simulink model "Prueba_PID"  (R2023b)
settings: Solver=VariableStepAuto  StartTime=0.0  StopTime=10  RelTol=1e-3
values from neighbouring files (symbols this model uses):
  K1 = (2*Ts*Kp + Ki*Ts^2 + 2*Kd)/(2*Ts)    (= 55.639105)    [PID_SystemIdentification.m]
  K2 = (Ki*Ts^2 - 2*Ts*Kp - 4*Kd)/(2*Ts)    (= -94.547095)    [PID_SystemIdentification.m]
  K3 = (2*Kd)/(2*Ts)    (= 42.1)    [PID_SystemIdentification.m]
settings Model: Creator=PC  LastModifiedBy=Ruben

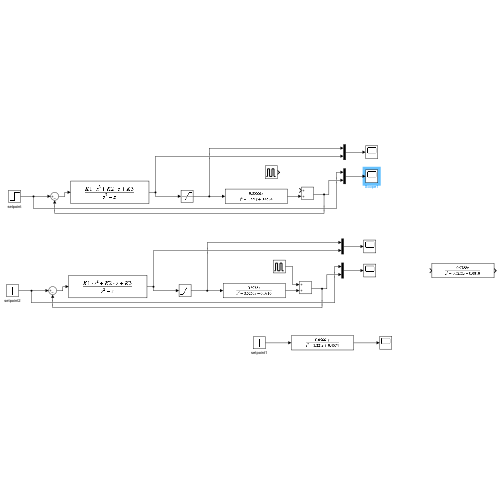
[thumbnail: Simulink's stored preview of the top-level diagram]
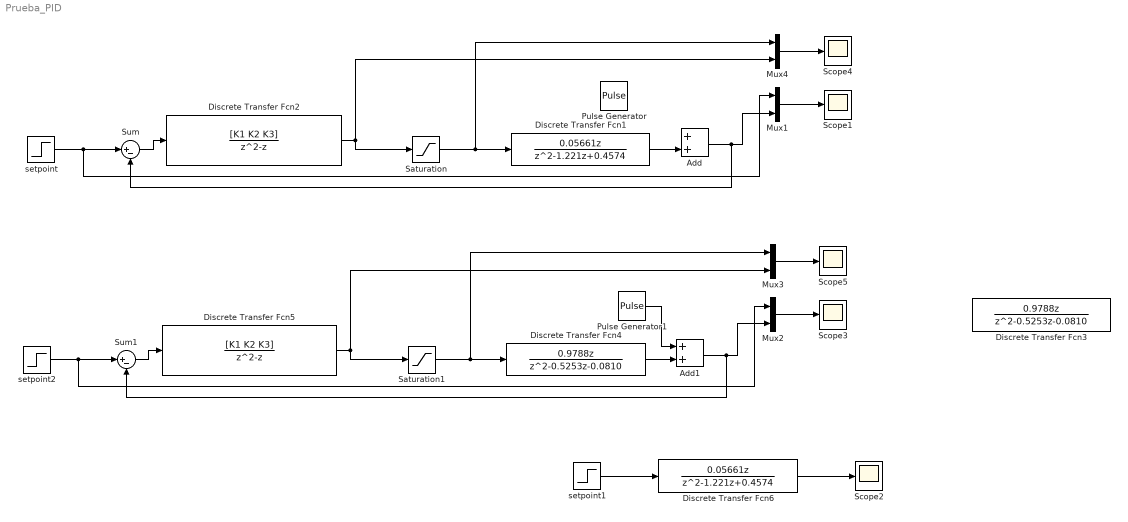
== system Prueba_PID ==
  Add : Sum
  Add1 : Sum
  Discrete Transfer Fcn1 : DiscreteTransferFcn  Numerator=[0.05661,0]  Denominator=[1,-1.221,0.4574]  SampleTime=0.1
  Discrete Transfer Fcn2 : DiscreteTransferFcn  Numerator=[K1 K2 K3]  Denominator=[1 -1 0]  SampleTime=0.031
  Discrete Transfer Fcn3 : DiscreteTransferFcn  Numerator=[0.9788, 0 ]  Denominator=[1,-0.5253,-0.0810]  SampleTime=0.031
  Discrete Transfer Fcn4 : DiscreteTransferFcn  Numerator=[0.9788, 0 ]  Denominator=[1,-0.5253,-0.0810]  SampleTime=0.031
  Discrete Transfer Fcn5 : DiscreteTransferFcn  Numerator=[K1 K2 K3]  Denominator=[1 -1 0]  SampleTime=0.031
  Discrete Transfer Fcn6 : DiscreteTransferFcn  Numerator=[0.05661,0]  Denominator=[1,-1.221,0.4574]  SampleTime=0.1
  Mux{1..4} (4 alike) : Mux  Inputs=2
  Pulse Generator : DiscretePulseGenerator  PulseType=Time based  Amplitude=-1  Period=10  PulseWidth=50  PhaseDelay=5
  Pulse Generator1 : DiscretePulseGenerator  PulseType=Time based  Amplitude=-1  Period=10  PulseWidth=50  PhaseDelay=5
  Saturation : Saturate  UpperLimit=55  LowerLimit=0
  Saturation1 : Saturate  UpperLimit=48  LowerLimit=0
  Scope{1..5} (5 alike) : Scope
  Sum : Sum  Inputs=|+-
  Sum1 : Sum  Inputs=|+-
  setpoint : Step  After=10  SampleTime=0.1
  setpoint1 : Step  After=50  SampleTime=0.1
  setpoint2 : Step  After=30  SampleTime=0.031
  wires:
  Mux1/1 -> Scope1/1
  Mux4/1 -> Scope4/1
  Discrete Transfer Fcn1/1 -> Add/2
  Add/1 -> Sum/2, Mux1/2
  setpoint/1 -> Mux1/1, Sum/1
  Sum/1 -> Discrete Transfer Fcn2/1
  Discrete Transfer Fcn2/1 -> Mux4/2, Saturation/1
  Saturation/1 -> Mux4/1, Discrete Transfer Fcn1/1
  Saturation1/1 -> Mux3/1, Discrete Transfer Fcn4/1
  Pulse Generator1/1 -> Add1/1
  Discrete Transfer Fcn4/1 -> Add1/2
  setpoint2/1 -> Mux2/1, Sum1/1
  Discrete Transfer Fcn5/1 -> Mux3/2, Saturation1/1
  Mux3/1 -> Scope5/1
  Add1/1 -> Sum1/2, Mux2/2
  Sum1/1 -> Discrete Transfer Fcn5/1
  Mux2/1 -> Scope3/1
  setpoint1/1 -> Discrete Transfer Fcn6/1
  Discrete Transfer Fcn6/1 -> Scope2/1
